simulink model "discrete_controlled_system"  (R2017a)
settings: Solver=VariableStepAuto  StartTime=0.0  StopTime=t_f  RelTol=1e-3
values from neighbouring files (symbols this model uses):
  A = double(subs(A_sym, symbs, vals))    [load_params.m]
  B = double(subs(B_sym, symbs, vals))    [load_params.m]
  C = double(subs(C_sym, symbs, vals))    [load_params.m]    (also in load_pwm_avg_pred_controller.m = sysd.c; load_pwm_pred_controller.m = sysd.c)
  Ctilde = double(subs(Ctilde_sym, symbs, vals))    [load_params.m]
  torque_ref = n_val*k_i_val*i_ref    [load_params.m]
  Ts_val = 1e-1    (= 0.1)    [load_params.m]    (also in load_pwm_controller.m; ss_value.m = 0.011)
  x0 = [0; 0]    [sim_controlled_system.m]
settings Model: Creator=brunolnetto  LastModifiedBy=brunolnetto

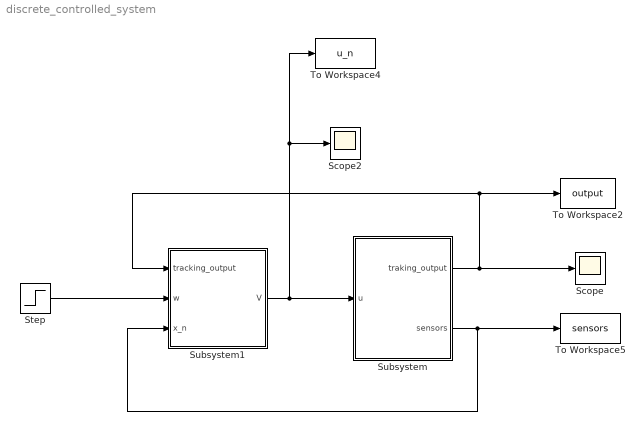
== system discrete_controlled_system ==
  Scope : Scope
  Scope2 : Scope
  Step : Step  Time=0  After=torque_ref  SampleTime=Ts_val
  Subsystem : Subsystem
  Subsystem1 : Subsystem
  To Workspace2 : ToWorkspace  VariableName=output  SaveFormat=Structure With Time  SampleTime=-1
  To Workspace4 : ToWorkspace  VariableName=u_n  SaveFormat=Structure With Time  SampleTime=-1
  To Workspace5 : ToWorkspace  VariableName=sensors  SaveFormat=Structure With Time  SampleTime=-1
  wires:
  Subsystem1/1(V) -> To Workspace4/1, Scope2/1, Subsystem/1(u)
  Subsystem/2(sensors) -> To Workspace5/1, Subsystem1/3(x_n)
  Subsystem/1(traking_output) -> Subsystem1/1(tracking_output), To Workspace2/1, Scope/1
  Step/1 -> Subsystem1/2(w)

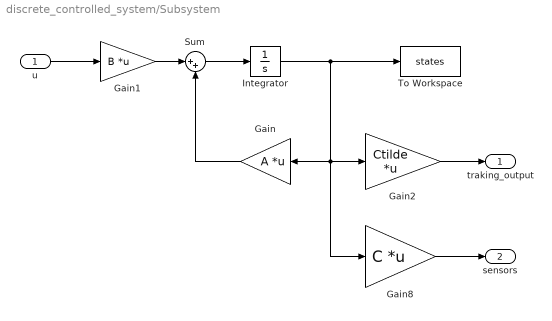
== system discrete_controlled_system/Subsystem ==
  u : Inport
  Gain : Gain  Gain=A  Multiplication=Matrix(K*u) (u vector)
  Gain1 : Gain  Gain=B  Multiplication=Matrix(K*u) (u vector)
  Gain2 : Gain  Gain=Ctilde  Multiplication=Matrix(K*u) (u vector)
  Gain8 : Gain  Gain=C  Multiplication=Matrix(K*u) (u vector)
  Integrator : Integrator  InitialCondition=x0
  Sum : Sum  Inputs=|++
  To Workspace : ToWorkspace  VariableName=states  SaveFormat=Structure With Time  SampleTime=-1
  traking_output : Outport
  sensors : Outport  Port=2
  wires:
  Gain8/1 -> sensors/1
  Gain1/1 -> Sum/1
  Integrator/1 -> To Workspace/1, Gain2/1, Gain8/1, Gain/1
  u/1 -> Gain1/1
  Gain/1 -> Sum/2
  Sum/1 -> Integrator/1
  Gain2/1 -> traking_output/1

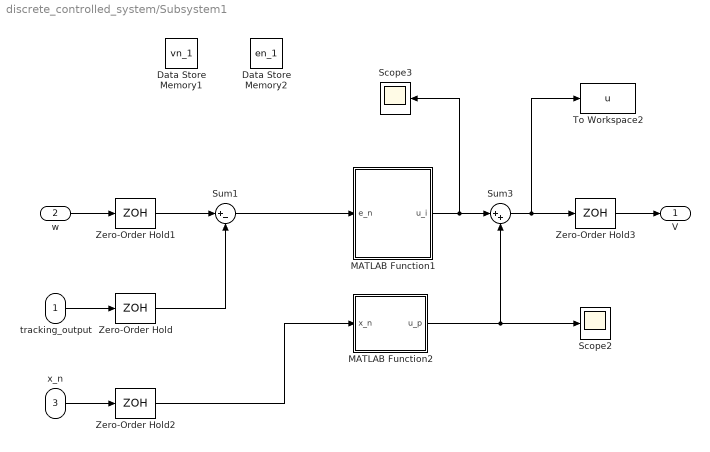
== system discrete_controlled_system/Subsystem1 ==
  tracking_output : Inport
  w : Inport  Port=2
  x_n : Inport  Port=3
  Data Store Memory1 : DataStoreMemory  DataStoreName=vn_1  ReadBeforeWriteMsg=warning  WriteAfterWriteMsg=warning  WriteAfterReadMsg=warning  ShowAdditionalParam=off  OutDataTypeStr=double
  Data Store Memory2 : DataStoreMemory  DataStoreName=en_1  ReadBeforeWriteMsg=warning  WriteAfterWriteMsg=warning  WriteAfterReadMsg=warning  InitialValue=e0  ShowAdditionalParam=off  OutDataTypeStr=double
  MATLAB Function1 : MATLAB Function  TreatAsAtomicUnit=on
  MATLAB Function2 : MATLAB Function  TreatAsAtomicUnit=on
  Scope2 : Scope
  Scope3 : Scope
  Sum1 : Sum  Inputs=|+-
  Sum3 : Sum  Inputs=|++
  To Workspace2 : ToWorkspace  VariableName=u  SaveFormat=Structure With Time  SampleTime=-1
  Zero-Order Hold{,1..3} (4 alike) : ZeroOrderHold  SampleTime=Ts_val
  V : Outport
  wires:
  tracking_output/1 -> Zero-Order Hold/1
  Zero-Order Hold2/1 -> MATLAB Function2/1(x_n)
  Sum3/1 -> To Workspace2/1, Zero-Order Hold3/1
  x_n/1 -> Zero-Order Hold2/1
  Zero-Order Hold/1 -> Sum1/2
  w/1 -> Zero-Order Hold1/1
  MATLAB Function2/1(u_p) -> Sum3/2, Scope2/1
  MATLAB Function1/1(u_i) -> Sum3/1, Scope3/1
  Zero-Order Hold1/1 -> Sum1/1
  Sum1/1 -> MATLAB Function1/1(e_n)
  Zero-Order Hold3/1 -> V/1

== matlab function discrete_controlled_system/Subsystem1/MATLAB Function2 ==
  data: x_n input; u_p output; params parameter
function u_p = proportional(x_n, params)
    u_p = - params.Kp*x_n;
end

== matlab function discrete_controlled_system/Subsystem1/MATLAB Function1 ==
  data: e_n input; u_i output; vn_1 data_store_memory; params parameter; en_1 data_store_memory
function u_i = integrator(e_n, params)
    global vn_1;
    global en_1;
    
    v_n = vn_1 + en_1;
    
    u_i = params.Ki*v_n;
    
    vn_1 = v_n;
    en_1 = e_n;
end
